simulink model "VirtualVehicleTemplate"  (R2023a)
settings: configuration reference "VehicleVariable" (kept outside this file)
StartFcn:
  | %tic
StopFcn:
  | %toc
undefined symbols (not defined in the file): CtrlEcuRevLim, CtrlTcuInitGear, CtrlVcuCltch1InitCmd, Disabled, DriverPreviewDist, EnvAbsPrs, EnvAirTemp, EnvGrvty, EnvNomFrictionScaling, EnvNominalGrade, EnvWindVelX, EnvWindVelY, EnvWindVelZ, FTP75, PlntVehDstCGFrntAxl, PlntVehDstCGRearAxl, PlntVehInitLatPos, PlntVehInitLongPos, PlntVehInitPitchAng, PlntVehInitRollAng, PlntVehInitVertPos, PlntVehInitYawAng, PlntVehMass, PlntVehTrckWdth, PlntVehYawMomentInertia, ScnCRMaxLatAccel, ScnCRRadius, ScnDLCGateLongPos, ScnDLCLatRef, ScnDLCLatRefOffset, ScnDLCLongRefBpt, ScnDLCLongRefStartPos, ScnDLCVehicleWidth, ScnFHCounterDwellTime, ScnFHInitialDwellTime, ScnFHReturnTime, ScnFHRollRateZeroCross, ScnFHSteerAmp, ScnFHSteerSpeed, ScnISHandwheelRate, ScnISMaxHandwheelAng, ScnISMaxLatAccel, ScnISSteerHoldTime, ScnLongVelRef, ScnSDDwellTime, ScnSDSteerAmp, ScnSDSteerFreq, ScnSimTime, ScnSSFinalFreq, ScnSSSteerAmp, ScnSSSweepTime, ScnStartTime
libraries: simulink x18, vehdynlibscenariocommon x7, vehdynlibviscommon x3, vehdynlibdriver x2, sim3dgroundtruthsensorlib x2, autolibshared x2, autolibsharedcommon x1, sharedtransform x1, sim3dlib x1, sim3dautolib x1
(part 2 of 5)

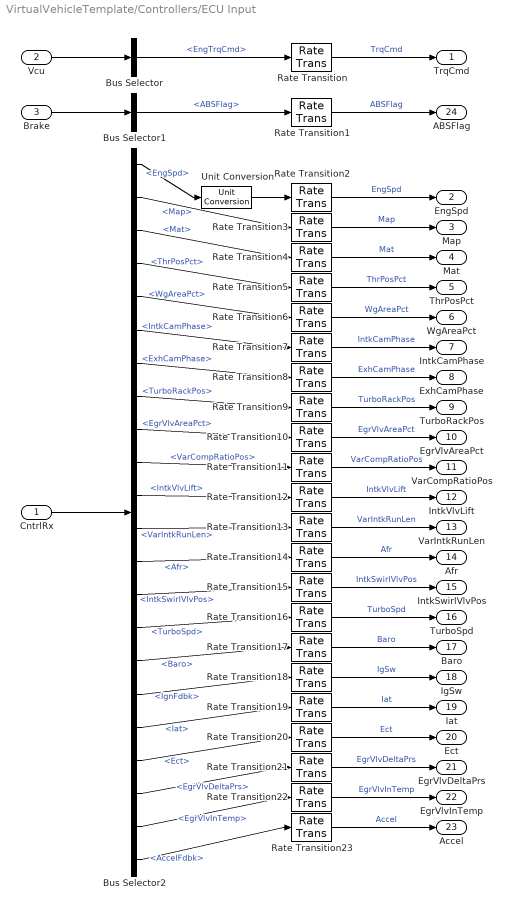
== system VirtualVehicleTemplate/Controllers/ECU Input ==
  CntrlRx : Inport
  Vcu : Inport  Port=2
  Brake : Inport  Port=3
  Bus Selector : BusSelector  OutputSignals=EngTrqCmd
  Bus Selector1 : BusSelector  OutputSignals=ABSFlag
  Bus Selector2 : BusSelector  OutputSignals=Trans.EngSpd,Engine.Map,Engine.Mat,Engine.ThrPosPct,Engine.WgAreaPct,Engine.IntkCamPhase,Engine.ExhCamPhase,Engine.TurboRackPos,Engine.EgrVlvAreaPct,Engine.VarCompRatioPos,Engine.IntkVlvLift,Engine.VarIntkRunLen,Engine.Afr,Engine.IntkSwirlVlvPos,Engine.TurboSpd,Env.Baro,Driver.IgnFdbk,Engine.Iat,Engine.Ect,Engine.EgrVlvDeltaPrs,Engine.EgrVlvInTemp,Driver.AccelFdbk
  Rate Transition{,1..23} (24 alike) : RateTransition  Deterministic=off
  Unit Conversion : UnitConversion
  TrqCmd : Outport
  EngSpd : Outport  Port=2
  Map : Outport  Port=3
  Mat : Outport  Port=4
  ThrPosPct : Outport  Port=5
  WgAreaPct : Outport  Port=6
  IntkCamPhase : Outport  Port=7
  ExhCamPhase : Outport  Port=8
  TurboRackPos : Outport  Port=9
  EgrVlvAreaPct : Outport  Port=10
  VarCompRatioPos : Outport  Port=11
  IntkVlvLift : Outport  Port=12
  VarIntkRunLen : Outport  Port=13
  Afr : Outport  Port=14
  IntkSwirlVlvPos : Outport  Port=15
  TurboSpd : Outport  Port=16
  Baro : Outport  Port=17
  IgSw : Outport  Port=18
  Iat : Outport  Port=19
  Ect : Outport  Port=20
  EgrVlvDeltaPrs : Outport  Port=21
  EgrVlvInTemp : Outport  Port=22
  Accel : Outport  Port=23
  ABSFlag : Outport  Port=24
  wires:
  Bus Selector2/13 -> Rate Transition14/1  "<Afr>"
  Bus Selector2/1 -> Unit Conversion/1  "<EngSpd>"
  Bus Selector2/21 -> Rate Transition22/1  "<EgrVlvInTemp>"
  Bus Selector2/19 -> Rate Transition20/1  "<Ect>"
  Bus Selector2/9 -> Rate Transition10/1  "<EgrVlvAreaPct>"
  Bus Selector2/15 -> Rate Transition16/1  "<TurboSpd>"
  Bus Selector2/17 -> Rate Transition18/1  "<IgnFdbk>"
  Bus Selector2/16 -> Rate Transition17/1  "<Baro>"
  Bus Selector2/2 -> Rate Transition3/1  "<Map>"
  Bus Selector2/18 -> Rate Transition19/1  "<Iat>"
  Bus Selector2/8 -> Rate Transition9/1  "<TurboRackPos>"
  Bus Selector2/10 -> Rate Transition11/1  "<VarCompRatioPos>"
  Bus Selector2/3 -> Rate Transition4/1  "<Mat>"
  Unit Conversion/1 -> Rate Transition2/1
  Bus Selector2/14 -> Rate Transition15/1  "<IntkSwirlVlvPos>"
  Bus Selector2/7 -> Rate Transition8/1  "<ExhCamPhase>"
  Bus Selector2/6 -> Rate Transition7/1  "<IntkCamPhase>"
  CntrlRx/1 -> Bus Selector2/1
  Bus Selector2/11 -> Rate Transition12/1  "<IntkVlvLift>"
  Bus Selector2/20 -> Rate Transition21/1  "<EgrVlvDeltaPrs>"
  Bus Selector2/12 -> Rate Transition13/1  "<VarIntkRunLen>"
  Bus Selector2/5 -> Rate Transition6/1  "<WgAreaPct>"
  Bus Selector2/4 -> Rate Transition5/1  "<ThrPosPct>"
  Bus Selector/1 -> Rate Transition/1  "<EngTrqCmd>"
  Vcu/1 -> Bus Selector/1
  Brake/1 -> Bus Selector1/1
  Bus Selector1/1 -> Rate Transition1/1  "<ABSFlag>"
  Bus Selector2/22 -> Rate Transition23/1  "<AccelFdbk>"
  Rate Transition/1 -> TrqCmd/1  "TrqCmd"
  Rate Transition1/1 -> ABSFlag/1  "ABSFlag"
  Rate Transition2/1 -> EngSpd/1  "EngSpd"
  Rate Transition3/1 -> Map/1  "Map"
  Rate Transition4/1 -> Mat/1  "Mat"
  Rate Transition5/1 -> ThrPosPct/1  "ThrPosPct"
  Rate Transition6/1 -> WgAreaPct/1  "WgAreaPct"
  Rate Transition7/1 -> IntkCamPhase/1  "IntkCamPhase"
  Rate Transition8/1 -> ExhCamPhase/1  "ExhCamPhase"
  Rate Transition9/1 -> TurboRackPos/1  "TurboRackPos"
  Rate Transition10/1 -> EgrVlvAreaPct/1  "EgrVlvAreaPct"
  Rate Transition11/1 -> VarCompRatioPos/1  "VarCompRatioPos"
  Rate Transition12/1 -> IntkVlvLift/1  "IntkVlvLift"
  Rate Transition13/1 -> VarIntkRunLen/1  "VarIntkRunLen"
  Rate Transition14/1 -> Afr/1  "Afr"
  Rate Transition15/1 -> IntkSwirlVlvPos/1  "IntkSwirlVlvPos"
  Rate Transition16/1 -> TurboSpd/1  "TurboSpd"
  Rate Transition17/1 -> Baro/1  "Baro"
  Rate Transition18/1 -> IgSw/1  "IgSw"
  Rate Transition19/1 -> Iat/1  "Iat"
  Rate Transition20/1 -> Ect/1  "Ect"
  Rate Transition21/1 -> EgrVlvDeltaPrs/1  "EgrVlvDeltaPrs"
  Rate Transition22/1 -> EgrVlvInTemp/1  "EgrVlvInTemp"
  Rate Transition23/1 -> Accel/1  "Accel"

== system VirtualVehicleTemplate/Controllers/ECU Output ==
  ThrPosPctCmd : Inport
  WgAreaPctCmd : Inport  Port=2
  InjPw : Inport  Port=3
  FuelMainSoi : Inport  Port=4
  SpkAdv : Inport  Port=5
  IntkCamPhaseCmd : Inport  Port=6
  ExhCamPhaseCmd : Inport  Port=7
  TurboRackPosCmd : Inport  Port=8
  EgrVlvAreaPctCmd : Inport  Port=9
  VarCompRatioPosCmd : Inport  Port=10
  IntkVlvLiftCmd : Inport  Port=11
  VarIntkRunLenCmd : Inport  Port=12
  ClsdLpFuelMult : Inport  Port=13
  IntkSwirlVlvPosCmd : Inport  Port=14
  TrqCmdISC : Inport  Port=15
  LoadCmd : Inport  Port=16
  EstIntkPortFlw : Inport  Port=17
  Bus Creator : BusCreator  Inputs=17
  Engine : Outport
  wires:
  Bus Creator/1 -> Engine/1  "Engine"
  EstIntkPortFlw/1 -> Bus Creator/17  "EstIntkPortFlw"
  ThrPosPctCmd/1 -> Bus Creator/1  "ThrPosPctCmd"
  InjPw/1 -> Bus Creator/3  "InjPw"
  SpkAdv/1 -> Bus Creator/5  "SpkAdv"
  TrqCmdISC/1 -> Bus Creator/15  "TrqCmd"
  VarCompRatioPosCmd/1 -> Bus Creator/10  "VarCompRatioPosCmd"
  FuelMainSoi/1 -> Bus Creator/4  "FuelMainSoi"
  IntkCamPhaseCmd/1 -> Bus Creator/6  "IntkCamPhaseCmd"
  ClsdLpFuelMult/1 -> Bus Creator/13  "ClsdLpFuelMult"
  WgAreaPctCmd/1 -> Bus Creator/2  "WgAreaPctCmd"
  ExhCamPhaseCmd/1 -> Bus Creator/7  "ExhCamPhaseCmd"
  TurboRackPosCmd/1 -> Bus Creator/8  "TurboRackPosCmd"
  EgrVlvAreaPctCmd/1 -> Bus Creator/9  "EgrVlvAreaPctCmd"
  IntkVlvLiftCmd/1 -> Bus Creator/11  "IntkVlvLiftCmd"
  VarIntkRunLenCmd/1 -> Bus Creator/12  "VarIntkRunLenCmd"
  IntkSwirlVlvPosCmd/1 -> Bus Creator/14  "IntkSwirlVlvPosCmd"
  LoadCmd/1 -> Bus Creator/16  "LoadCmd"

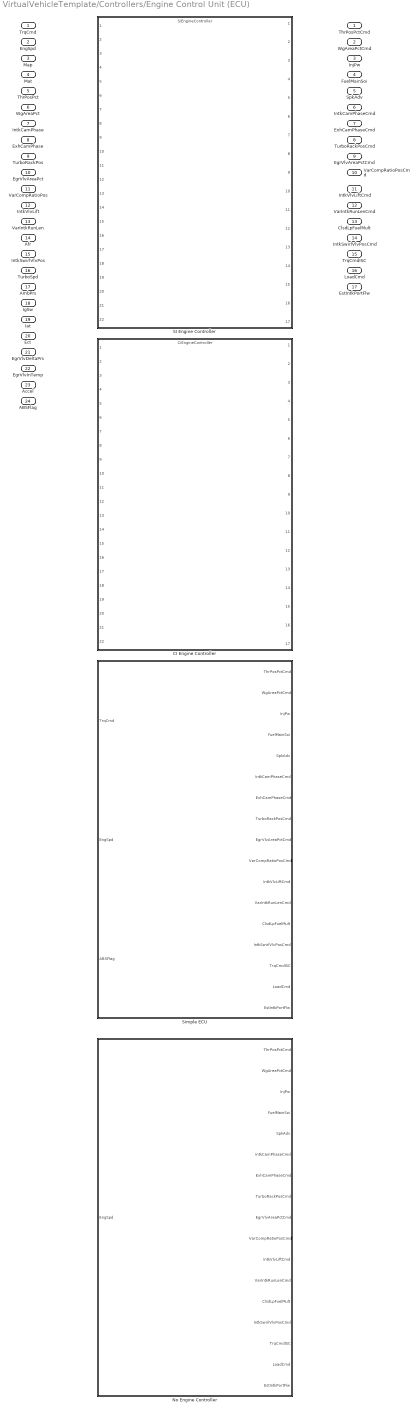
== system VirtualVehicleTemplate/Controllers/Engine Control Unit (ECU) ==
  TrqCmd : Inport
  EngSpd : Inport  Port=2
  Map : Inport  Port=3
  Mat : Inport  Port=4
  ThrPosPct : Inport  Port=5
  WgAreaPct : Inport  Port=6
  IntkCamPhase : Inport  Port=7
  ExhCamPhase : Inport  Port=8
  TurboRackPos : Inport  Port=9
  EgrVlvAreaPct : Inport  Port=10
  VarCompRatioPos : Inport  Port=11
  IntkVlvLift : Inport  Port=12
  VarIntkRunLen : Inport  Port=13
  Afr : Inport  Port=14
  IntkSwirlVlvPos : Inport  Port=15
  TurboSpd : Inport  Port=16
  AmbPrs : Inport  Port=17
  IgSw : Inport  Port=18
  Iat : Inport  Port=19
  Ect : Inport  Port=20
  EgrVlvDeltaPrs : Inport  Port=21
  EgrVlvInTemp : Inport  Port=22
  Accel : Inport  Port=23
  ABSFlag : Inport  Port=24
  CI Engine Controller : ModelReference  ModelNameDialog=CiEngineController  SimulationMode=Normal  VariantControl=CI Engine Controller  ModelReferenceVersion=7.0
  No Engine Controller : Subsystem  VariantControl=No Engine Controller
  SI Engine Controller : ModelReference  ModelNameDialog=SiEngineController  SimulationMode=Normal  VariantControl=SI Engine Controller  ModelReferenceVersion=6.2
  Simple ECU : Subsystem  VariantControl=Simple ECU
  ThrPosPctCmd : Outport  VectorParamsAs1DForOutWhenUnconnected=off
  WgAreaPctCmd : Outport  Port=2  VectorParamsAs1DForOutWhenUnconnected=off
  InjPw : Outport  Port=3  VectorParamsAs1DForOutWhenUnconnected=off
  FuelMainSoi : Outport  Port=4  VectorParamsAs1DForOutWhenUnconnected=off
  SpkAdv : Outport  Port=5  VectorParamsAs1DForOutWhenUnconnected=off
  IntkCamPhaseCmd : Outport  Port=6  VectorParamsAs1DForOutWhenUnconnected=off
  ExhCamPhaseCmd : Outport  Port=7  VectorParamsAs1DForOutWhenUnconnected=off
  TurboRackPosCmd : Outport  Port=8  VectorParamsAs1DForOutWhenUnconnected=off
  EgrVlvAreaPctCmd : Outport  Port=9  VectorParamsAs1DForOutWhenUnconnected=off
  VarCompRatioPosCmd : Outport  Port=10  VectorParamsAs1DForOutWhenUnconnected=off
  IntkVlvLiftCmd : Outport  Port=11  VectorParamsAs1DForOutWhenUnconnected=off
  VarIntkRunLenCmd : Outport  Port=12  VectorParamsAs1DForOutWhenUnconnected=off
  ClsdLpFuelMult : Outport  Port=13  VectorParamsAs1DForOutWhenUnconnected=off
  IntkSwirlVlvPosCmd : Outport  Port=14  VectorParamsAs1DForOutWhenUnconnected=off
  TrqCmdISC : Outport  Port=15  VectorParamsAs1DForOutWhenUnconnected=off
  LoadCmd : Outport  Port=16  VectorParamsAs1DForOutWhenUnconnected=off
  EstIntkPortFlw : Outport  Port=17  VectorParamsAs1DForOutWhenUnconnected=off

== system VirtualVehicleTemplate/Controllers/TCU Input ==
  CntrlRx : Inport
  Brake : Inport  Port=2
  Bus Selector : BusSelector  OutputSignals=ABSFlag
  Bus Selector1 : BusSelector  OutputSignals=Driver.AccelFdbk,Driver.DecelFdbk,Driver.GearFdbk,Trans.EngSpd,Wheels.Omega,Vehicle
  Ground : Ground
  Ground1 : Ground
  Rate Transition{1..8,23} (9 alike) : RateTransition  Deterministic=off
  <AccFdbk> : Outport
  <DecelFdbk> : Outport  Port=2
  <GearFdbk> : Outport  Port=3
  <EngSpd> : Outport  Port=4
  <Omega> : Outport  Port=5
  <Vehicle> : Outport  Port=6
  ABSFlag : Outport  Port=7
  UpReq : Outport  Port=8
  DnReq : Outport  Port=9
  wires:
  Bus Selector1/6 -> Rate Transition5/1  "<Vehicle>"
  Bus Selector1/2 -> Rate Transition1/1  "<DecelFdbk>"
  Ground/1 -> Rate Transition7/1
  CntrlRx/1 -> Bus Selector1/1
  Bus Selector1/1 -> Rate Transition23/1  "<AccelFdbk>"
  Bus Selector1/5 -> Rate Transition4/1  "<Omega>"
  Bus Selector1/4 -> Rate Transition3/1  "<EngSpd>"
  Bus Selector1/3 -> Rate Transition2/1  "<GearFdbk>"
  Ground1/1 -> Rate Transition8/1
  Bus Selector/1 -> Rate Transition6/1  "<ABSFlag>"
  Brake/1 -> Bus Selector/1
  Rate Transition23/1 -> <AccFdbk>/1
  Rate Transition1/1 -> <DecelFdbk>/1
  Rate Transition2/1 -> <GearFdbk>/1
  Rate Transition3/1 -> <EngSpd>/1
  Rate Transition4/1 -> <Omega>/1
  Rate Transition5/1 -> <Vehicle>/1
  Rate Transition6/1 -> ABSFlag/1
  Rate Transition7/1 -> UpReq/1
  Rate Transition8/1 -> DnReq/1

== system VirtualVehicleTemplate/Controllers/TCU Output ==
  GearCmd : Inport
  Bus Creator1 : BusCreator  Inputs=1
  Trans : Outport
  wires:
  Bus Creator1/1 -> Trans/1  "Trans"
  GearCmd/1 -> Bus Creator1/1  "GearCmd"

== system VirtualVehicleTemplate/Controllers/Transmission Control Unit (TCU) ==
  Accel : Inport
  BrkCmd : Inport  Port=2
  GearReq : Inport  Port=3
  EngSpd : Inport  Port=4
  Omega : Inport  Port=5  Unit=rad/s
  VehSpdFdbk : Inport  Port=6
  ABSFlag : Inport  Port=7
  UpReq : Inport  Port=8
  DownReq : Inport  Port=9  Unit=rad/s
  Driver Pass Through : ModelReference  ModelNameDialog=DriverPassThrough.slx  VariantControl=Driver Pass Through  ModelReferenceVersion=6.0
  Transmission Controller : ModelReference  ModelNameDialog=TransmissionController  VariantControl=PRNDL Controller  ModelReferenceVersion=6.0
  " Gear" : Outport  VectorParamsAs1DForOutWhenUnconnected=off

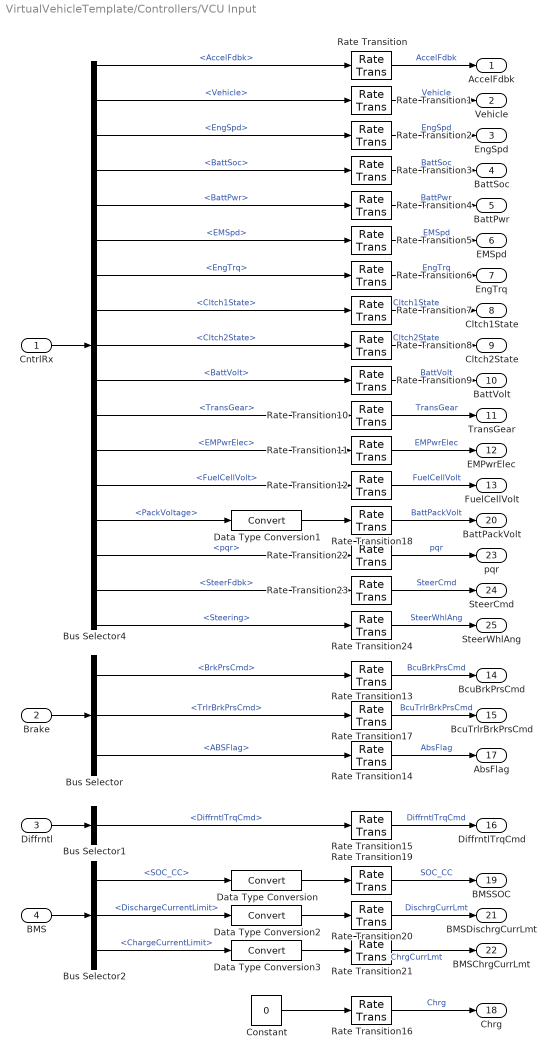
== system VirtualVehicleTemplate/Controllers/VCU Input ==
  CntrlRx : Inport
  Brake : Inport  Port=2
  Diffrntl : Inport  Port=3
  BMS : Inport  Port=4
  Bus Selector : BusSelector  OutputSignals=BrkPrsCmd,TrlrBrkPrsCmd,ABSFlag
  Bus Selector1 : BusSelector  OutputSignals=DiffrntlTrqCmd
  Bus Selector2 : BusSelector  OutputSignals=BMSInfo.SOC.SOC_CC,BMSCmd.CurrentLimitsBus.DischargeCurrentLimit,BMSCmd.CurrentLimitsBus.ChargeCurrentLimit
  Bus Selector4 : BusSelector  OutputSignals=Driver.AccelFdbk,Vehicle,Trans.EngSpd,Battery.BattSoc,Battery.BattPwr,Trans.EMSpd,Engine.EngTrq,Trans.Cltch1State,Trans.Cltch2State,Battery.BattVolt,Trans.TransGear,EM.EMPwrElec,FuelCell.FuelCellVolt,Battery.BMSSensors.PackVoltage,IMU.pqr,Driver.SteerFdbk,Steering
  Constant : Constant  Value=0  SampleTime=-1
  Data Type Conversion{,1..3} (4 alike) : DataTypeConversion  SaturateOnIntegerOverflow=off  RndMeth=Floor
  Rate Transition{,1..24} (25 alike) : RateTransition  Deterministic=off
  AccelFdbk : Outport
  Vehicle : Outport  Port=2
  EngSpd : Outport  Port=3
  BattSoc : Outport  Port=4
  BattPwr : Outport  Port=5
  EMSpd : Outport  Port=6
  EngTrq : Outport  Port=7
  Cltch1State : Outport  Port=8
  Cltch2State : Outport  Port=9
  BattVolt : Outport  Port=10
  TransGear : Outport  Port=11
  EMPwrElec : Outport  Port=12
  FuelCellVolt : Outport  Port=13
  BcuBrkPrsCmd : Outport  Port=14
  BcuTrlrBrkPrsCmd : Outport  Port=15
  DiffrntlTrqCmd : Outport  Port=16
  AbsFlag : Outport  Port=17
  Chrg : Outport  Port=18
  BMSSOC : Outport  Port=19
  BattPackVolt : Outport  Port=20
  BMSDischrgCurrLmt : Outport  Port=21
  BMSChrgCurrLmt : Outport  Port=22
  pqr : Outport  Port=23
  SteerCmd : Outport  Port=24
  SteerWhlAng : Outport  Port=25
  wires:
  Bus Selector4/5 -> Rate Transition4/1  "<BattPwr>"
  Bus Selector4/1 -> Rate Transition/1  "<AccelFdbk>"
  Bus Selector4/7 -> Rate Transition6/1  "<EngTrq>"
  Bus Selector4/4 -> Rate Transition3/1  "<BattSoc>"
  Bus Selector4/6 -> Rate Transition5/1  "<EMSpd>"
  CntrlRx/1 -> Bus Selector4/1
  Bus Selector4/11 -> Rate Transition10/1  "<TransGear>"
  Bus Selector4/9 -> Rate Transition8/1  "<Cltch2State>"
  Bus Selector4/13 -> Rate Transition12/1  "<FuelCellVolt>"
  Bus Selector4/2 -> Rate Transition1/1  "<Vehicle>"
  Bus Selector4/8 -> Rate Transition7/1  "<Cltch1State>"
  Bus Selector4/10 -> Rate Transition9/1  "<BattVolt>"
  Bus Selector4/3 -> Rate Transition2/1  "<EngSpd>"
  Bus Selector4/12 -> Rate Transition11/1  "<EMPwrElec>"
  Bus Selector/1 -> Rate Transition13/1  "<BrkPrsCmd>"
  Constant/1 -> Rate Transition16/1
  Brake/1 -> Bus Selector/1
  Bus Selector/3 -> Rate Transition14/1  "<ABSFlag>"
  Diffrntl/1 -> Bus Selector1/1
  Bus Selector1/1 -> Rate Transition15/1  "<DiffrntlTrqCmd>"
  Rate Transition/1 -> AccelFdbk/1  "AccelFdbk"
  Rate Transition1/1 -> Vehicle/1  "Vehicle"
  Rate Transition2/1 -> EngSpd/1  "EngSpd"
  Rate Transition3/1 -> BattSoc/1  "BattSoc"
  Rate Transition4/1 -> BattPwr/1  "BattPwr"
  Rate Transition5/1 -> EMSpd/1  "EMSpd"
  Rate Transition6/1 -> EngTrq/1  "EngTrq"
  Rate Transition7/1 -> Cltch1State/1  "Cltch1State"
  Rate Transition8/1 -> Cltch2State/1  "Cltch2State"
  Rate Transition9/1 -> BattVolt/1  "BattVolt"
  Rate Transition10/1 -> TransGear/1  "TransGear"
  Rate Transition11/1 -> EMPwrElec/1  "EMPwrElec"
  Rate Transition12/1 -> FuelCellVolt/1  "FuelCellVolt"
  Rate Transition13/1 -> BcuBrkPrsCmd/1  "BcuBrkPrsCmd"
  Rate Transition14/1 -> AbsFlag/1  "AbsFlag"
  Rate Transition15/1 -> DiffrntlTrqCmd/1  "DiffrntlTrqCmd"
  Rate Transition16/1 -> Chrg/1  "Chrg"
  Rate Transition20/1 -> BMSDischrgCurrLmt/1  "DischrgCurrLmt"
  Rate Transition19/1 -> BMSSOC/1  "SOC_CC"
  Rate Transition21/1 -> BMSChrgCurrLmt/1  "ChrgCurrLmt"
  Data Type Conversion3/1 -> Rate Transition21/1
  Data Type Conversion2/1 -> Rate Transition20/1
  Bus Selector2/1 -> Data Type Conversion/1  "<SOC_CC>"
  Data Type Conversion/1 -> Rate Transition19/1
  Bus Selector2/3 -> Data Type Conversion3/1  "<ChargeCurrentLimit>"
  Bus Selector2/2 -> Data Type Conversion2/1  "<DischargeCurrentLimit>"
  BMS/1 -> Bus Selector2/1
  Data Type Conversion1/1 -> Rate Transition18/1
  Rate Transition18/1 -> BattPackVolt/1  "BattPackVolt"
  Bus Selector4/14 -> Data Type Conversion1/1  "<PackVoltage>"
  Bus Selector/2 -> Rate Transition17/1  "<TrlrBrkPrsCmd>"
  Rate Transition17/1 -> BcuTrlrBrkPrsCmd/1  "BcuTrlrBrkPrsCmd"
  Rate Transition22/1 -> pqr/1  "pqr"
  Rate Transition23/1 -> SteerCmd/1  "SteerCmd"
  Rate Transition24/1 -> SteerWhlAng/1  "SteerWhlAng"
  Bus Selector4/15 -> Rate Transition22/1  "<pqr>"
  Bus Selector4/16 -> Rate Transition23/1  "<SteerFdbk>"
  Bus Selector4/17 -> Rate Transition24/1  "<Steering>"

== system VirtualVehicleTemplate/Controllers/VCU Output ==
  EngTrqCmd : Inport
  EMTrqCmd : Inport  Port=2
  VcuBrkPrsCmd : Inport  Port=3
  VcuTrlrBrkPrsCmd : Inport  Port=4
  Cltch1Cmd : Inport  Port=5
  Neutral : Inport  Port=6
  FuelCellCurrCmd : Inport  Port=7
  FuelCellTempCmd : Inport  Port=8
  Bus Creator5 : BusCreator  Inputs=8
  Vcu : Outport
  wires:
  Cltch1Cmd/1 -> Bus Creator5/5  "Cltch1Cmd"
  EngTrqCmd/1 -> Bus Creator5/1  "EngTrqCmd"
  Bus Creator5/1 -> Vcu/1  "Vcu"
  VcuBrkPrsCmd/1 -> Bus Creator5/3  "VcuBrkPrsCmd"
  Neutral/1 -> Bus Creator5/6  "Neutral"
  FuelCellCurrCmd/1 -> Bus Creator5/7  "FuelCellCurrCmd"
  EMTrqCmd/1 -> Bus Creator5/2  "EMTrqCmd"
  FuelCellTempCmd/1 -> Bus Creator5/8  "FuelCellTempCmd"
  VcuTrlrBrkPrsCmd/1 -> Bus Creator5/4  "VcuTrlrBrkPrsCmd"

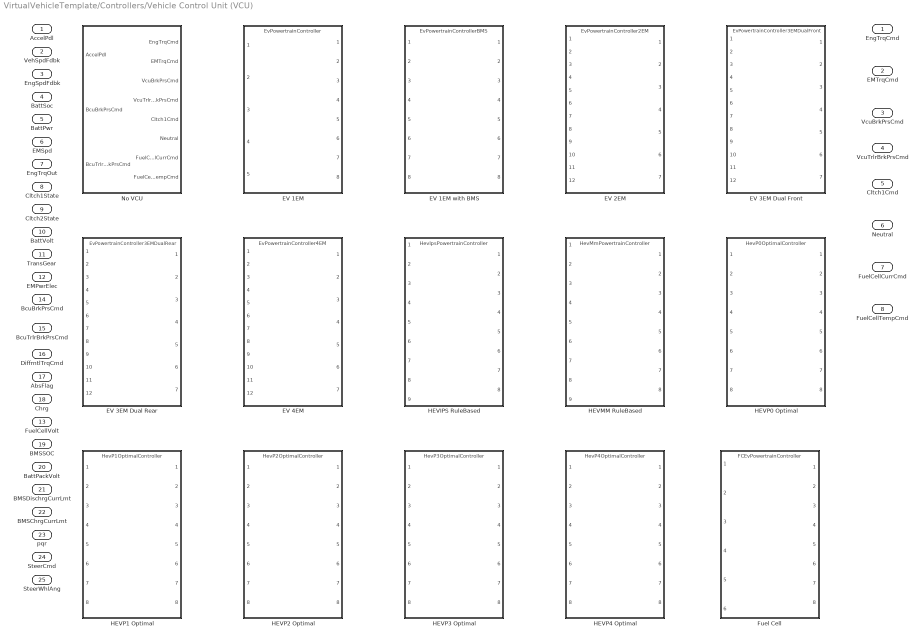
== system VirtualVehicleTemplate/Controllers/Vehicle Control Unit (VCU) ==
  AccelPdl : Inport
  VehSpdFdbk : Inport  Port=2
  EngSpdFdbk : Inport  Port=3
  BattSoc : Inport  Port=4
  BattPwr : Inport  Port=5
  EMSpd : Inport  Port=6
  EngTrqOut : Inport  Port=7
  Cltch1State : Inport  Port=8
  Cltch2State : Inport  Port=9
  BattVolt : Inport  Port=10
  TransGear : Inport  Port=11
  EMPwrElec : Inport  Port=12
  FuelCellVolt : Inport  Port=13
  BcuBrkPrsCmd : Inport  Port=14
  BcuTrlrBrkPrsCmd : Inport  Port=15
  DiffrntlTrqCmd : Inport  Port=16
  AbsFlag : Inport  Port=17
  Chrg : Inport  Port=18
  BMSSOC : Inport  Port=19
  BattPackVolt : Inport  Port=20
  BMSDischrgCurrLmt : Inport  Port=21
  BMSChrgCurrLmt : Inport  Port=22
  pqr : Inport  Port=23
  SteerCmd : Inport  Port=24
  SteerWhlAng : Inport  Port=25
  EV 1EM : ModelReference  ModelNameDialog=EvPowertrainController  VariantControl=EV 1EM  ModelReferenceVersion=6.24
  EV 1EM with BMS : ModelReference  ModelNameDialog=EvPowertrainControllerBMS.slx  VariantControl=EV 1EM with BMS  ModelReferenceVersion=6.17
  EV 2EM : ModelReference  ModelNameDialog=EvPowertrainController2EM.slx  VariantControl=EV 2EM  ModelReferenceVersion=6.43
  EV 3EM Dual Front : ModelReference  ModelNameDialog=EvPowertrainController3EMDualFront.slx  VariantControl=EV 3EM Dual Front  ModelReferenceVersion=6.44
  EV 3EM Dual Rear : ModelReference  ModelNameDialog=EvPowertrainController3EMDualRear.slx  VariantControl=EV 3EM Dual Rear  ModelReferenceVersion=6.43
  EV 4EM : ModelReference  ModelNameDialog=EvPowertrainController4EM.slx  VariantControl=EV 4EM  ModelReferenceVersion=6.46
  Fuel Cell : ModelReference  ModelNameDialog=FCEvPowertrainController  VariantControl=Fuel Cell  ModelReferenceVersion=6.12
  HEVIPS RuleBased : ModelReference  ModelNameDialog=HevIpsPowertrainController  VariantControl=HEVIPS RuleBased  ModelReferenceVersion=11.16
  HEVMM RuleBased : ModelReference  ModelNameDialog=HevMmPowertrainController  VariantControl=HEVMM RuleBased  ModelReferenceVersion=11.15
  HEVP0 Optimal : ModelReference  ModelNameDialog=HevP0OptimalController  VariantControl=HEVP0 Optimal  ModelReferenceVersion=6.17
  HEVP1 Optimal : ModelReference  ModelNameDialog=HevP1OptimalController  VariantControl=HEVP1 Optimal  ModelReferenceVersion=6.13
  HEVP2 Optimal : ModelReference  ModelNameDialog=HevP2OptimalController  VariantControl=HEVP2 Optimal  ModelReferenceVersion=6.14
  HEVP3 Optimal : ModelReference  ModelNameDialog=HevP3OptimalController  VariantControl=HEVP3 Optimal  ModelReferenceVersion=6.13
  HEVP4 Optimal : ModelReference  ModelNameDialog=HevP4OptimalController  VariantControl=HEVP4 Optimal  ModelReferenceVersion=6.13
  No VCU : Subsystem  SystemSampleTime=.01  VariantControl=No VCU
  EngTrqCmd : Outport  VectorParamsAs1DForOutWhenUnconnected=off
  EMTrqCmd : Outport  Port=2  VectorParamsAs1DForOutWhenUnconnected=off
  VcuBrkPrsCmd : Outport  Port=3  VectorParamsAs1DForOutWhenUnconnected=off
  VcuTrlrBrkPrsCmd : Outport  Port=4  VectorParamsAs1DForOutWhenUnconnected=off
  Cltch1Cmd : Outport  Port=5  VectorParamsAs1DForOutWhenUnconnected=off
  Neutral : Outport  Port=6  VectorParamsAs1DForOutWhenUnconnected=off
  FuelCellCurrCmd : Outport  Port=7  VectorParamsAs1DForOutWhenUnconnected=off
  FuelCellTempCmd : Outport  Port=8  VectorParamsAs1DForOutWhenUnconnected=off

== system VirtualVehicleTemplate/Driver Commands/Driver Commands ==
  VehRef : Inport
  VehFdbk : Inport  Port=2
  Env : Inport  Port=3
  SteerCmd : Inport  Port=4
  AccelCmd : Inport  Port=5
  BrakeCmd : Inport  Port=6
  GearCmd : Inport  Port=7
  Longitudinal Driver : Subsystem  VariantControl=driverType==1
  Open Loop : Subsystem  VariantControl=driverType==4
  Predictive Driver : Subsystem  VariantControl=driverType==2
  Predictive Stanley Driver : Subsystem  VariantControl=driverType==3
  " Driver" : Outport  VectorParamsAs1DForOutWhenUnconnected=off

== system VirtualVehicleTemplate/Environment/Estimated Grade ==
  Gnd : Inport
  Atan : Trigonometry  Operator=atan
  Bus Selector : BusSelector  OutputSignals=z  OutputAsBus=on
  Bus to Vector : BusToVector
  Constant Grade : Constant  Value=EnvNominalGrade  SampleTime=-1
  Constant1 : Constant  Value=PlntVehDstCGFrntAxl+PlntVehDstCGRearAxl  SampleTime=-1
  Divide : Product  Inputs=*/
  Gain : Gain  Gain=.5
  Gain1 : Gain  Gain=.5
  Grade Source : ManualSwitch  CurrentSetting=0
  Selector : Selector  InputPortWidth=4  IndexOptions=Index vector (dialog)  Indices=[1 2]  OutputSizes=1
  Selector1 : Selector  InputPortWidth=4  IndexOptions=Index vector (dialog)  Indices=[3 4]  OutputSizes=1
  Signal Specification : SignalSpecification  Unit=rad
  Signal Specification1 : SignalSpecification  Unit=deg
  Signal Specification2 : SignalSpecification  Unit=deg
  Subtract : Sum  Inputs=+-
  Sum of Elements : Sum  Inputs=+
  Sum of Elements1 : Sum  Inputs=+
  Unit Conversion : UnitConversion
  Grade : Outport  PortDimensions=1
  wires:
  Divide/1 -> Atan/1
  Bus Selector/1 -> Bus to Vector/1
  Sum of Elements/1 -> Gain/1
  Gain/1 -> Subtract/1
  Selector/1 -> Sum of Elements/1
  Sum of Elements1/1 -> Gain1/1
  Signal Specification/1 -> Unit Conversion/1
  Constant1/1 -> Divide/2
  Selector1/1 -> Sum of Elements1/1
  Gain1/1 -> Subtract/2
  Subtract/1 -> Divide/1
  Atan/1 -> Signal Specification/1
  Grade Source/1 -> Grade/1  "Grade"
  Gnd/1 -> Bus Selector/1
  Bus to Vector/1 -> Selector1/1, Selector/1
  Constant Grade/1 -> Signal Specification2/1
  Signal Specification2/1 -> Grade Source/2
  Unit Conversion/1 -> Signal Specification1/1
  Signal Specification1/1 -> Grade Source/1  "Grade"

== system VirtualVehicleTemplate/Environment/Ground Feedback ==
  Friction : Inport
  WheelFdbk : Inport  Port=2
  3D Engine : Subsystem  VariantControl=1
  Constant : Subsystem  VariantControl=0
  Ground : Outport  VectorParamsAs1DForOutWhenUnconnected=off

== system VirtualVehicleTemplate/Environment/Varying Friction ==
  In1 : Inport
  In2 : Inport  Port=2
  Cg : Inport  Port=3
  Constant Friction : Subsystem  VariantControl=0
  Varying Friction : Subsystem  VariantControl=1
  FricCoeffLambda : Outport

== system VirtualVehicleTemplate/Scenarios/Drive Cycle ==
  "VehFdbk " : Inport
  Bus Creator : BusCreator  Inputs=3
  Bus Creator1 : BusCreator  Inputs=16
  Constant{,2..3,8,13..15,17} (8 alike) : Constant  Value=0
  Constant{1,4..7,9..12} (9 alike) : Constant  Value=false
  Constant16 : Constant  Value=zeros(1,3)
  Drive Cycle Source : autolibshared/Drive Cycle Source  cycleVar=FTP75  fileVar=L:\Bauto\matlab\test\toolbox\shared\autoblks\scenario\adac.txt  tfinal="2474  seconds"  cycleRepeat=off  outAccPort=off  outGearPort=off  gearList=No gear data  t_wot1=1  xdot_woto=0  xdot_wot1=26.8  t_wot2=30  xdot_wot2=0  t_wotend=40  srcUnit=m/s  outUnit=mph  srcAccUnit=m/s/s  outAccUnit=m/s^2  dt=0  aMode=6  faultOption=off  velBnd=2  velBndUnit=mph  inUnit=m/s  timeBnd=1  failOption=off  stopSim=off  maxFaultCnt=10  maxFaultTime=2  maxTotFaultTime=15  traceOption=off  dtTrace=1  traceWindow=10  lastDCname=FTP75  lastOutUnit=mph  lastDT=0  lastTB=1  lastSB=2  forceCalcBound=off
  Signal Specification : SignalSpecification  Unit=rad
  Signal Specification1 : SignalSpecification  Unit=one
  Signal Specification2 : SignalSpecification  Unit=one
  " Vis" : Outport  VectorParamsAs1DForOutWhenUnconnected=off
  " Ref" : Outport  Port=2  VectorParamsAs1DForOutWhenUnconnected=off
  " Fdbk" : Outport  Port=3  VectorParamsAs1DForOutWhenUnconnected=off
  wires:
  Constant2/1 -> Signal Specification2/1
  Constant8/1 -> Signal Specification1/1
  Constant4/1 -> Bus Creator1/7  "SteerHld"
  Signal Specification2/1 -> Bus Creator1/14  "DecelOvrCmd"
  Constant12/1 -> Bus Creator1/16  "DecelZero"
  Constant6/1 -> Bus Creator1/9  "EnblAccelOvr"
  Constant7/1 -> Bus Creator1/11  "AccelHld"
  Constant9/1 -> Bus Creator1/12  "AccelZero"
  Signal Specification1/1 -> Bus Creator1/10  "AccelOvrCmd"
  Constant11/1 -> Bus Creator1/15  "DecelHld"
  Constant10/1 -> Bus Creator1/13  "EnblDecelCmd"
  Constant5/1 -> Bus Creator1/8  "SteerZero"
  Signal Specification/1 -> Bus Creator1/6  "SteerOvrCmd"
  Constant3/1 -> Signal Specification/1
  Constant1/1 -> Bus Creator1/5  "EnblSteerCmd"
  Constant/1 -> Bus Creator1/2  "LtrlRef"
  Drive Cycle Source/1 -> Bus Creator1/1  "LngRef"
  Bus Creator1/1 -> " Ref"/1
  "VehFdbk "/1 -> " Fdbk"/1
  Bus Creator/1 -> " Vis"/1
  Constant15/1 -> Bus Creator/3  "ZRef"
  Constant14/1 -> Bus Creator/2  "YRef"
  Constant13/1 -> Bus Creator/1  "XRef"
  Constant16/1 -> Bus Creator1/3  "PoseRef"
  Constant17/1 -> Bus Creator1/4  "CurvRef"

== system VirtualVehicleTemplate/Scenarios/Reference Generator ==
  "VehFdbk " : Inport
  3D Engine : Subsystem  Variant=on  mask(3D Engine){engine3D=Disabled, SceneDesc=Open surface, dt3D=dt3D, defaultPos=Recommended for scene, X_o=X_o, Y_o=Y_o, Z_o=Z_o, phi_o=phi_o, theta_o=theta_o, psi_o=psi_o}
      mask prompts: engine3D "3D Engine"; SceneDesc "shared_sim3dblks:sim3dblkConfig:SceneDesc"; dt3D "Engine frame rate, dt3D [s]:"; X_o "Initial longitudinal position, X_o [m]:"; Y_o "Initial lateral position, Y_o [m]:"; Z_o "Initial vertical position, Z_o [m]:"; phi_o "Initial roll angle, phi_o [rad]:"; theta_o "Initial pitch angle, theta_o [rad]:"; psi_o "Initial yaw angle, psi_o [rad]:"
      mask help: This subsystem contains the interface blocks which permit the display of the vehicle in the 3D virtual environment. Enable it to view the simulation progress, disable it to inhibit the display.
      mask init:
      | GrndFdbkPath = [bdroot(gcb) '/Environment/Ground Feedback'];
      | switch get_param(gcb,'engine3D')    
      |     case 'Disabled'
      |         try
      |             set_param(GrndFdbkPath,'LabelModeActiveChoice','0');
      |             set_param([bdroot(gcb) '/Scenarios/Reference Generator/Reference Generator/Double Lane Change/Double Lane Change'],'use3DCones','off');
      |             set_param([bdroot(gcb) '/Scenarios/Reference Generator/Reference Generator/Constant Radius'],'use3DCones','off');
      |         catch
      |             disp('Warning: Ground feedback source subsystem was not found. Ground feedback source remains unchanged.');
      |         end
      |     case 'Enabled'
      |         try
      |             set_param(GrndFdbkPath,'LabelModeActiveChoice','1'); 
      |             set_param([bdroot(gcb) '/Scenarios/Reference Generator/Reference Generator/Double Lane Change/Double Lane Change'],'use3DCones','on');
      |             set_param([bdroot(gcb) '/Scenarios/Reference Generator/Reference Generator/Constant Radius'],'use3DCones','on');
      |         catch
      |             disp('Warning: Ground feedback source subsystem was not found. Ground feedback source remains unchanged.');
      |         end
      |     otherwise
      | end
      settings: AttributesFormatString=|
      | %<SceneDesc>
      | %<engine3D>
      mask Help: eval('vdynblkshelp(''vdynblks3dengine'')');
      mask TypeOptions engine3D: vdynblks:vehdynRefApp3DEng:blkRdBt_engine3D_c2 | vdynblks:vehdynRefApp3DEng:blkRdBt_engine3D_c1
      mask TypeOptions SceneDesc: 3D Engine/Simulation 3D Scene Configuration/SceneDesc
      mask Callback SceneDesc: [~] = vdynblks3Dsceneconfig(gcb);
      mask TypeOptions defaultPos: vdynblks:vehdynRefApp3DEng:blkRdBt_defaultPos_c1 | vdynblks:vehdynRefApp3DEng:blkRdBt_defaultPos_c2
      mask DialogControl engineConfig Prompt: 3D Engine Settings
      mask DialogControl SceneDesc Prompt: Scene name:
      mask DialogControl posSetup Prompt: Initial vehicle position
      mask DialogControl posSetupDesc Prompt: To use these initial vehicle positions, first Apply the initial values and then click Update the model workspaces with the initial values.
      mask DialogControl setModelPos Prompt: Update model workspaces with initial values
      mask DialogControl setModelPos Callback: [~] = vdynblksmdlWSconfig(gcb);
      mask Display: disp('3D Engine')
  Reference Generator : Subsystem  Variant=on  VariantControlMode=label  VariantControl=Variant1  LabelModeActiveChoice=Drive Cycle
  " Vis" : Outport  VectorParamsAs1DForOutWhenUnconnected=off
  " Ref" : Outport  Port=2  VectorParamsAs1DForOutWhenUnconnected=off
  " Fdbk" : Outport  Port=3  VectorParamsAs1DForOutWhenUnconnected=off
  wires:
  Reference Generator/3(" Fdbk") -> " Fdbk"/1
  Reference Generator/2(" Ref") -> " Ref"/1
  Reference Generator/1(" Vis") -> " Vis"/1
  "VehFdbk "/1 -> Reference Generator/1("VehFdbk "), 3D Engine/1(VehFdbk)

== system VirtualVehicleTemplate/Vehicle/Chassis Input ==
  Env : Inport
  Driver : Inport  Port=2
  Cntrl : Inport  Port=3
  Bus Selector1 : BusSelector  OutputSignals=Gnd.z.G_FL_z,Gnd.z.G_FR_z,Gnd.z.G_RL_z,Gnd.z.G_RR_z
  Bus Selector2 : BusSelector  OutputSignals=Wind
  Bus Selector3 : BusSelector  OutputSignals=Gnd.mu.mu_FL,Gnd.mu.mu_FR,Gnd.mu.mu_RL,Gnd.mu.mu_RR
  Bus Selector4 : BusSelector  OutputSignals=Grade
  Bus Selector5 : BusSelector  OutputSignals=SteerCmd
  Bus Selector6 : BusSelector  OutputSignals=Vcu.VcuBrkPrsCmd
  Bus Selector7 : BusSelector  OutputSignals=Gnd.DCM
  First Order Hold1 : FirstOrderHold  ErrorTolerance=inf
  Vector Concatenate : Concatenate  NumInputs=4
  Vector Concatenate1 : Concatenate  NumInputs=4
  Wind : Outport  VectorParamsAs1DForOutWhenUnconnected=off
  Gnd : Outport  Port=2  VectorParamsAs1DForOutWhenUnconnected=off
  Mu : Outport  Port=3  VectorParamsAs1DForOutWhenUnconnected=off
  Grade : Outport  Port=4  VectorParamsAs1DForOutWhenUnconnected=off
  GndDCM : Outport  Port=5  VectorParamsAs1DForOutWhenUnconnected=off
  SteerCmd : Outport  Port=6  VectorParamsAs1DForOutWhenUnconnected=off
  BrkPrsCmd : Outport  Port=7  VectorParamsAs1DForOutWhenUnconnected=off
  wires:
  Env/1 -> Bus Selector7/1, Bus Selector4/1, Bus Selector3/1, Bus Selector1/1, Bus Selector2/1
  Bus Selector2/1 -> Wind/1  "<Wind>"
  Bus Selector3/1 -> Vector Concatenate/1  "<mu_FL>"
  Bus Selector3/2 -> Vector Concatenate/2  "<mu_FR>"
  Bus Selector3/3 -> Vector Concatenate/3  "<mu_RL>"
  Bus Selector3/4 -> Vector Concatenate/4  "<mu_RR>"
  Vector Concatenate/1 -> Mu/1
  Bus Selector1/1 -> Vector Concatenate1/1  "<G_FL_z>"
  Bus Selector1/2 -> Vector Concatenate1/2  "<G_FR_z>"
  Bus Selector1/3 -> Vector Concatenate1/3  "<G_RL_z>"
  Bus Selector1/4 -> Vector Concatenate1/4  "<G_RR_z>"
  Vector Concatenate1/1 -> Gnd/1
  Driver/1 -> Bus Selector5/1
  Bus Selector5/1 -> SteerCmd/1  "<SteerCmd>"
  Cntrl/1 -> Bus Selector6/1
  Bus Selector6/1 -> First Order Hold1/1  "<VcuBrkPrsCmd>"
  Bus Selector4/1 -> Grade/1  "<Grade>"
  First Order Hold1/1 -> BrkPrsCmd/1
  Bus Selector7/1 -> GndDCM/1  "<DCM>"

== system VirtualVehicleTemplate/Vehicle/Chassis Output ==
  Veh : Inport
  Wheels : Inport  Port=2
  Steering : Inport  Port=3
  Susp : Inport  Port=4
  Out Bus Element4 : Outport  PortName=VehFdbk
  Out Bus Element1 : Outport  Port=2  PortName=WheelsFdbk
  Out Bus Element2 : Outport  Port=3  PortName=SteeringFdbk
  Out Bus Element3 : Outport  Port=4  PortName=SuspensionFdbk
  wires:
  Veh/1 -> Out Bus Element4/1
  Wheels/1 -> Out Bus Element1/1
  Steering/1 -> Out Bus Element2/1
  Susp/1 -> Out Bus Element3/1

== system VirtualVehicleTemplate/Vehicle/Drivetrain Input ==
  Cntrl : Inport
  Bus Selector3 : BusSelector  OutputSignals=Trans.GearCmd,Vcu.Cltch1Cmd,Diff.DiffrntlPrsCmd
  First Order Hold1 : FirstOrderHold  ErrorTolerance=inf
  Rate Transition : RateTransition  InitialCondition=CtrlTcuInitGear
  Rate Transition1 : RateTransition  InitialCondition=CtrlVcuCltch1InitCmd
  GearCmd : Outport  VectorParamsAs1DForOutWhenUnconnected=off
  Cltch1Cmd : Outport  Port=2  VectorParamsAs1DForOutWhenUnconnected=off
  DiffrntlPrsCmd : Outport  Port=3  VectorParamsAs1DForOutWhenUnconnected=off
  wires:
  Cntrl/1 -> Bus Selector3/1
  Bus Selector3/1 -> Rate Transition/1  "<GearCmd>"
  Bus Selector3/3 -> First Order Hold1/1  "<DiffrntlPrsCmd>"
  Bus Selector3/2 -> Rate Transition1/1  "<Cltch1Cmd>"
  Rate Transition1/1 -> Cltch1Cmd/1
  First Order Hold1/1 -> DiffrntlPrsCmd/1
  Rate Transition/1 -> GearCmd/1

== system VirtualVehicleTemplate/Vehicle/Drivetrain Output ==
  AxlTrq : Inport
  EngSpd : Inport  Port=2
  DriveshftSpd : Inport  Port=3
  EMSpd : Inport  Port=4
  TransInfo : Inport  Port=5
  Bus Creator1 : BusCreator  Inputs=5
  Driveline : Outport  VectorParamsAs1DForOutWhenUnconnected=off
  wires:
  Bus Creator1/1 -> Driveline/1  "Driveline"
  DriveshftSpd/1 -> Bus Creator1/3  "DriveshftSpd"
  AxlTrq/1 -> Bus Creator1/1  "AxlTrq"
  EngSpd/1 -> Bus Creator1/2  "EngSpd"
  EMSpd/1 -> Bus Creator1/4  "EMSpd"
  TransInfo/1 -> Bus Creator1/5  "TransInfo"

== system VirtualVehicleTemplate/Vehicle/Electrical System Input ==
  Cntrl : Inport
  Env : Inport  Port=2
  Bus Selector : BusSelector  OutputSignals=Temp
  Bus Selector2 : BusSelector  OutputSignals=Vcu.EMTrqCmd,Vcu.FuelCellCurrCmd,Vcu.FuelCellTempCmd,BMS
  First Order Hold : FirstOrderHold  ErrorTolerance=inf  AllowContinuousInput=on
  First Order Hold1 : FirstOrderHold  ErrorTolerance=inf  AllowContinuousInput=on
  First Order Hold2 : FirstOrderHold  ErrorTolerance=inf  AllowContinuousInput=on
  EMTrqCmd : Outport  VectorParamsAs1DForOutWhenUnconnected=off
  AmbTemp : Outport  Port=2  VectorParamsAs1DForOutWhenUnconnected=off
  FuelCellCurrCmd : Outport  Port=3  VectorParamsAs1DForOutWhenUnconnected=off
  FuelCellTempCmd : Outport  Port=4  VectorParamsAs1DForOutWhenUnconnected=off
  BMS : Outport  Port=5  VectorParamsAs1DForOutWhenUnconnected=off
  wires:
  Env/1 -> Bus Selector/1
  Bus Selector/1 -> AmbTemp/1  "<Temp>"
  Cntrl/1 -> Bus Selector2/1
  Bus Selector2/1 -> First Order Hold/1  "<EMTrqCmd>"
  First Order Hold/1 -> EMTrqCmd/1  "EMTrqCmd"
  First Order Hold1/1 -> FuelCellCurrCmd/1  "FuelCellCurrCmd"
  First Order Hold2/1 -> FuelCellTempCmd/1  "FuelCellTempCmd"
  Bus Selector2/2 -> First Order Hold1/1  "<FuelCellCurrCmd>"
  Bus Selector2/3 -> First Order Hold2/1  "<FuelCellTempCmd>"
  Bus Selector2/4 -> BMS/1  "<BMS>"

== system VirtualVehicleTemplate/Vehicle/Electrical System Output ==
  Battery : Inport
  ElecMachine : Inport  Port=2
  FuelCell : Inport  Port=3
  Out Bus Element4 : Outport  PortName=BatteryFdbk
  Out Bus Element1 : Outport  Port=2  PortName=ElecMachineFdbk
  Out Bus Element2 : Outport  Port=3  PortName=FuelCellFdbk
  wires:
  Battery/1 -> Out Bus Element4/1
  ElecMachine/1 -> Out Bus Element1/1
  FuelCell/1 -> Out Bus Element2/1

== system VirtualVehicleTemplate/Vehicle/Engine Input ==
  Cntrl : Inport
  Bus Creator : BusCreator  Inputs=17
  Bus Selector : BusSelector  OutputSignals=Engine.ThrPosPctCmd,Engine.WgAreaPctCmd,Engine.InjPw,Engine.FuelMainSoi,Engine.SpkAdv,Engine.IntkCamPhaseCmd,Engine.ExhCamPhaseCmd,Engine.TurboRackPosCmd,Engine.EgrVlvAreaPctCmd,Engine.VarCompRatioPosCmd,Engine.IntkVlvLiftCmd,Engine.VarIntkRunLenCmd,Engine.ClsdLpFuelMult,Engine.IntkSwirlVlvPosCmd,Engine.TrqCmd,Engine.LoadCmd,Engine.EstIntkPortFlw
  First Order Hold{,1..16} (17 alike) : FirstOrderHold  ErrorTolerance=inf
  Engine : Outport
  wires:
  Bus Selector/14 -> First Order Hold14/1  "<IntkSwirlVlvPosCmd>"
  Bus Selector/12 -> First Order Hold13/1  "<VarIntkRunLenCmd>"
  Bus Selector/15 -> First Order Hold2/1  "<TrqCmd>"
  Bus Selector/13 -> First Order Hold/1  "<ClsdLpFuelMult>"
  Bus Selector/7 -> First Order Hold8/1  "<ExhCamPhaseCmd>"
  First Order Hold11/1 -> Bus Creator/10  "VarCompRatioPosCmd"
  Bus Selector/4 -> First Order Hold3/1  "<FuelMainSoi>"
  Bus Selector/8 -> First Order Hold9/1  "<TurboRackPosCmd>"
  Bus Selector/5 -> First Order Hold4/1  "<SpkAdv>"
  Bus Selector/9 -> First Order Hold10/1  "<EgrVlvAreaPctCmd>"
  Bus Selector/11 -> First Order Hold12/1  "<IntkVlvLiftCmd>"
  First Order Hold/1 -> Bus Creator/13  "ClsdLpFuelMult"
  Bus Selector/6 -> First Order Hold7/1  "<IntkCamPhaseCmd>"
  First Order Hold1/1 -> Bus Creator/3  "InjPw"
  First Order Hold7/1 -> Bus Creator/6  "IntkCamPhaseCmd"
  First Order Hold9/1 -> Bus Creator/8  "TurboRackPosCmd"
  Bus Selector/3 -> First Order Hold1/1  "<InjPw>"
  First Order Hold5/1 -> Bus Creator/1  "ThrPosPctCmd"
  First Order Hold3/1 -> Bus Creator/4  "FuelMainSoi"
  First Order Hold10/1 -> Bus Creator/9  "EgrVlvAreaPctCmd"
  First Order Hold12/1 -> Bus Creator/11  "IntkVlvLiftCmd"
  First Order Hold13/1 -> Bus Creator/12  "VarIntkRunLenCmd"
  First Order Hold2/1 -> Bus Creator/15  "TrqCmd"
  Bus Selector/1 -> First Order Hold5/1  "<ThrPosPctCmd>"
  Bus Selector/2 -> First Order Hold6/1  "<WgAreaPctCmd>"
  First Order Hold8/1 -> Bus Creator/7  "ExhCamPhaseCmd"
  First Order Hold6/1 -> Bus Creator/2  "WgAreaPctCmd"
  First Order Hold14/1 -> Bus Creator/14  "IntkSwirlVlvPosCmd"
  First Order Hold4/1 -> Bus Creator/5  "SpkAdv"
  Bus Selector/10 -> First Order Hold11/1  "<VarCompRatioPosCmd>"
  Bus Creator/1 -> Engine/1  "Engine"
  Cntrl/1 -> Bus Selector/1
  Bus Selector/16 -> First Order Hold15/1  "<LoadCmd>"
  Bus Selector/17 -> First Order Hold16/1  "<EstIntkPortFlw>"
  First Order Hold15/1 -> Bus Creator/16  "LoadCmd"
  First Order Hold16/1 -> Bus Creator/17  "EstIntkPortFlw"

== system VirtualVehicleTemplate/Vehicle/Engine Output ==
  "EngFdbk " : Inport
  EngFdbk : Outport  VectorParamsAs1DForOutWhenUnconnected=off
  wires:
  "EngFdbk "/1 -> EngFdbk/1  "EngFdbk"

== system VirtualVehicleTemplate/Vehicle/Pedal Cluster Input ==
  Driver : Inport
  Bus Selector : BusSelector  OutputSignals=SteerCmd,AccelCmd,DecelCmd,GearCmd,IgnSwtch
  SteerCmd : Outport  VectorParamsAs1DForOutWhenUnconnected=off
  AccelCmd : Outport  Port=2  VectorParamsAs1DForOutWhenUnconnected=off
  DecelCmd : Outport  Port=3  VectorParamsAs1DForOutWhenUnconnected=off
  DrvrGearCmd : Outport  Port=4  VectorParamsAs1DForOutWhenUnconnected=off
  IgnCmd : Outport  Port=5  VectorParamsAs1DForOutWhenUnconnected=off
  wires:
  Bus Selector/2 -> AccelCmd/1  "<AccelCmd>"
  Driver/1 -> Bus Selector/1
  Bus Selector/3 -> DecelCmd/1  "<DecelCmd>"
  Bus Selector/4 -> DrvrGearCmd/1  "<GearCmd>"
  Bus Selector/1 -> SteerCmd/1  "<SteerCmd>"
  Bus Selector/5 -> IgnCmd/1  "<IgnSwtch>"

== system VirtualVehicleTemplate/Vehicle/Pedal Cluster Output ==
  Driver : Inport
  OperatorFdbk : Outport
  wires:
  Driver/1 -> OperatorFdbk/1

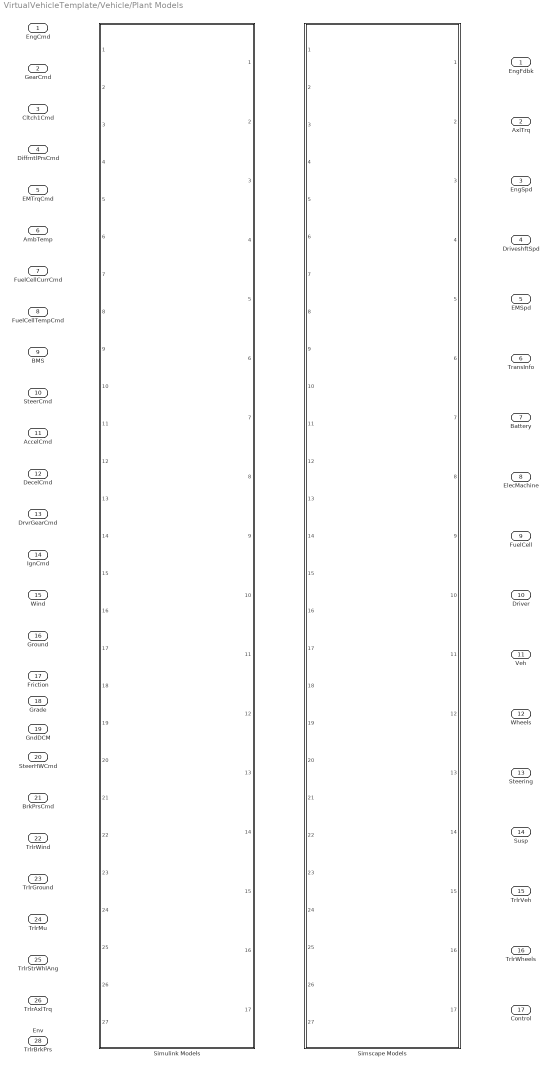
== system VirtualVehicleTemplate/Vehicle/Plant Models ==
  EngCmd : Inport
  GearCmd : Inport  Port=2
  Cltch1Cmd : Inport  Port=3
  DiffrntlPrsCmd : Inport  Port=4
  EMTrqCmd : Inport  Port=5
  AmbTemp : Inport  Port=6
  FuelCellCurrCmd : Inport  Port=7
  FuelCellTempCmd : Inport  Port=8
  BMS : Inport  Port=9
  SteerCmd : Inport  Port=10
  AccelCmd : Inport  Port=11
  DecelCmd : Inport  Port=12
  DrvrGearCmd : Inport  Port=13
  IgnCmd : Inport  Port=14
  Wind : Inport  Port=15
  Ground : Inport  Port=16
  Friction : Inport  Port=17
  Grade : Inport  Port=18
  GndDCM : Inport  Port=19
  SteerHWCmd : Inport  Port=20
  BrkPrsCmd : Inport  Port=21
  TrlrWind : Inport  Port=22
  TrlrGround : Inport  Port=23
  TrlrMu : Inport  Port=24
  TrlrStrWhlAng : Inport  Port=25
  TrlrAxlTrq : Inport  Port=26
  TrlrBrkPrs : Inport  Port=27
  Env : Inport  Port=28
  Simscape Models : Subsystem  VariantControl=SimscapeModels  ReferencedSubsystem=SimscapePlantModels
  Simulink Models : Subsystem  VariantControl=SimulinkModels  ReferencedSubsystem=SimulinkPlantModels
  EngFdbk : Outport
  AxlTrq : Outport  Port=2
  EngSpd : Outport  Port=3
  DriveshftSpd : Outport  Port=4
  EMSpd : Outport  Port=5
  TransInfo : Outport  Port=6
  Battery : Outport  Port=7
  ElecMachine : Outport  Port=8
  FuelCell : Outport  Port=9
  Driver : Outport  Port=10
  Veh : Outport  Port=11
  Wheels : Outport  Port=12
  Steering : Outport  Port=13
  Susp : Outport  Port=14
  TrlrVeh : Outport  Port=15
  TrlrWheels : Outport  Port=16
  Control : Outport  Port=17

== system VirtualVehicleTemplate/Vehicle/Sensor Input ==
  EnvIn : Inport
  Env : Outport
  wires:
  EnvIn/1 -> Env/1  "Env"

== system VirtualVehicleTemplate/Vehicle/Sensor Output ==
  Control : Inport
  CntrlFdbk : Outport
  wires:
  Control/1 -> CntrlFdbk/1

== system VirtualVehicleTemplate/Vehicle/Trailer Input ==
  Env : Inport
  Cntrl : Inport  Port=2
  Bus Selector2 : BusSelector  OutputSignals=Wind
  Bus Selector4 : BusSelector  OutputSignals=Vcu.VcuTrlrBrkPrsCmd
  Constant1 : Constant  Value=zeros(2,1)
  Constant2 : Constant  Value=ones(2,1)
  Constant3 : Constant  Value=[0 0 0 0 0 0]
  Constant4 : Constant  Value=0
  Ground Info Trailer : Subsystem  Commented=on  Variant=on  VariantControlMode=label  VariantControl=Choice  LabelModeActiveChoice=0
  Terminator1 : Terminator
  Terminator2 : Terminator
  TrlrWind : Outport  VectorParamsAs1DForOutWhenUnconnected=off
  TrlrGnd : Outport  Port=2  VectorParamsAs1DForOutWhenUnconnected=off
  TrlrMu : Outport  Port=3  VectorParamsAs1DForOutWhenUnconnected=off
  TrlrStrWhlAng : Outport  Port=4  VectorParamsAs1DForOutWhenUnconnected=off
  TrlrAxlTrq : Outport  Port=5  VectorParamsAs1DForOutWhenUnconnected=off
  TrlrBrkPrs : Outport  Port=6  VectorParamsAs1DForOutWhenUnconnected=off
  wires:
  Bus Selector2/1 -> TrlrWind/1  "<Wind>"
  Env/1 -> Bus Selector2/1, Ground Info Trailer/1(Env)
  Constant3/1 -> TrlrStrWhlAng/1
  Constant4/1 -> TrlrAxlTrq/1
  Bus Selector4/1 -> TrlrBrkPrs/1  "<VcuTrlrBrkPrsCmd>"
  Cntrl/1 -> Bus Selector4/1
  Constant2/1 -> TrlrMu/1
  Constant1/1 -> TrlrGnd/1
  Ground Info Trailer/1(Ground) -> Terminator1/1
  Ground Info Trailer/2(Friction) -> Terminator2/1

== system VirtualVehicleTemplate/Vehicle/Trailer Output ==
  Veh : Inport
  Wheels : Inport  Port=2
  Out Bus Element4 : Outport  PortName=VehFdbk
  Out Bus Element1 : Outport  Port=2  PortName=WheelsFdbk
  wires:
  Wheels/1 -> Out Bus Element1/1
  Veh/1 -> Out Bus Element4/1

== system VirtualVehicleTemplate/Visualization/DataLogging ==
  VehFdbk : Inport
  Bus Selector : BusSelector  OutputSignals=Driver.SteerFdbk
  Terminator : Terminator
  wires:
  VehFdbk/1 -> Bus Selector/1
  Bus Selector/1 -> Terminator/1  "<SteerFdbk>"

== system VirtualVehicleTemplate/Visualization/Emission Calculations ==
  VehSpd : Inport
  TP HC Mass Flow : Inport  Port=2
  TP CO Mass Flow : Inport  Port=3
  TP NOx Mass Flow : Inport  Port=4
  TP CO2 Mass Flow : Inport  Port=5
  Integrator{,1..4} (5 alike) : Integrator
  Kg to g : Gain  Gain=1000
  "Kg to g " : Gain  Gain=1000
  "Kg to g  " : Gain  Gain=1000
  "Kg to g   " : Gain  Gain=1000
  L/100 Km Calc{,1..3} (4 alike) : Product  Inputs=/*
  Rate Transition{,1..3} (4 alike) : RateTransition  Deterministic=off
  Saturation : Saturate  UpperLimit=Inf  LowerLimit=0.2  ZeroCross=off
  Saturation1 : Saturate  UpperLimit=Inf  LowerLimit=1  ZeroCross=off
  Signal Specification5 : SignalSpecification  Unit=m/s
  Unit Conversion5 : UnitConversion
  m to km : Gain  Gain=0.001
  m to mi : Gain  Gain=0.000621371
  TP HC Mass : Outport  VectorParamsAs1DForOutWhenUnconnected=off
  TP CO Mass : Outport  Port=2  VectorParamsAs1DForOutWhenUnconnected=off
  TP NOx Mass : Outport  Port=3  VectorParamsAs1DForOutWhenUnconnected=off
  TP CO2 Mass : Outport  Port=4  VectorParamsAs1DForOutWhenUnconnected=off
  wires:
  L/100 Km Calc/1 -> Rate Transition/1
  m to mi/1 -> Saturation/1
  Saturation/1 -> L/100 Km Calc2/1, L/100 Km Calc1/1, L/100 Km Calc/1
  TP HC Mass Flow/1 -> Integrator1/1
  Integrator1/1 -> Kg to g/1
  Integrator/1 -> m to km/1, m to mi/1
  Kg to g/1 -> L/100 Km Calc/2
  TP CO Mass Flow/1 -> Integrator2/1
  Integrator2/1 -> "Kg to g "/1
  "Kg to g "/1 -> L/100 Km Calc1/2
  TP NOx Mass Flow/1 -> Integrator3/1
  Integrator3/1 -> "Kg to g  "/1
  "Kg to g  "/1 -> L/100 Km Calc2/2
  L/100 Km Calc1/1 -> Rate Transition1/1
  L/100 Km Calc2/1 -> Rate Transition2/1
  TP CO2 Mass Flow/1 -> Integrator4/1
  Integrator4/1 -> "Kg to g   "/1
  "Kg to g   "/1 -> L/100 Km Calc3/2
  L/100 Km Calc3/1 -> Rate Transition3/1
  Saturation1/1 -> L/100 Km Calc3/1
  m to km/1 -> Saturation1/1
  Rate Transition/1 -> TP HC Mass/1  "TP HC Mass (g/mi)"
  Rate Transition1/1 -> TP CO Mass/1  "TP CO Mass (g/mi)"
  Rate Transition2/1 -> TP NOx Mass/1  "TP NOx Mass (g/mi)"
  Rate Transition3/1 -> TP CO2 Mass/1  "TP CO2 Mass (g/km)"
  Unit Conversion5/1 -> Signal Specification5/1
  VehSpd/1 -> Unit Conversion5/1
  Signal Specification5/1 -> Integrator/1

== system VirtualVehicleTemplate/Visualization/ISO 15037-1:2006 ==
  VehFdbk : Inport
  Disabled : Subsystem  VariantControl=0
  Enabled : Subsystem  VariantControl=1

== system VirtualVehicleTemplate/Visualization/Performance Calculations ==
  VehSpd : Inport
  FuelVolFlow : Inport  Port=2
  BattPwr : Inport  Port=3
  Add : Sum
  Divide : Product  Inputs=*/
  Divide1 : Product  Inputs=*/
  Divide2 : Product  Inputs=*/
  Integrator : Integrator
  Integrator1 : Integrator
  L/100 Km Calc : Product  Inputs=/*
  Product : Product
  Rate Transition3 : RateTransition  Deterministic=off
  Saturation : Saturate  UpperLimit=Inf  LowerLimit=0.001  ZeroCross=off
  Saturation1 : Saturate  UpperLimit=Inf  LowerLimit=1e-3  ZeroCross=off
  Signal Specification5 : SignalSpecification  Unit=m/s
  Sqrt : Sqrt
  US EPA kwh/USgal equivalent : Constant  Value=33.7
  US MPG Calc : Product  Inputs=*/
  Unit Conversion5 : UnitConversion
  m to 100Km : Gain  Gain=1/1000/100
  m to mile : Gain  Gain=0.000621371
  m^3 per gal : Gain  Gain=0.00378541
  m^3 to L : Gain  Gain=1000
  m^3 to US Gal : Gain  Gain=264.172
  s per h : Constant  Value=3600
  w per kw : Constant  Value=1000
  US MPG : Outport  VectorParamsAs1DForOutWhenUnconnected=off
  L/100Km : Outport  Port=2  VectorParamsAs1DForOutWhenUnconnected=off
  wires:
  m^3 to US Gal/1 -> Saturation1/1
  m^3 to L/1 -> L/100 Km Calc/2
  Integrator/1 -> m to mile/1, m to 100Km/1
  m to mile/1 -> US MPG Calc/1
  FuelVolFlow/1 -> Add/1
  Integrator1/1 -> m^3 to US Gal/1, m^3 to L/1
  Saturation/1 -> L/100 Km Calc/1
  m to 100Km/1 -> Saturation/1
  L/100 Km Calc/1 -> L/100Km/1  "L/100Km"
  US MPG Calc/1 -> Rate Transition3/1
  Saturation1/1 -> US MPG Calc/2
  Rate Transition3/1 -> US MPG/1  "US MPG"
  w per kw/1 -> Divide/2
  Divide/1 -> Divide2/1
  Divide2/1 -> Divide1/1
  s per h/1 -> Divide1/2
  Divide1/1 -> m^3 per gal/1
  Add/1 -> Integrator1/1
  m^3 per gal/1 -> Add/2
  US EPA kwh/USgal equivalent/1 -> Divide2/2
  BattPwr/1 -> Divide/1
  Sqrt/1 -> Integrator/1
  Product/1 -> Sqrt/1
  Signal Specification5/1 -> Product/2, Product/1
  Unit Conversion5/1 -> Signal Specification5/1
  VehSpd/1 -> Unit Conversion5/1

== system VirtualVehicleTemplate/Visualization/Scope Type ==
  "VehFdbk " : Inport
  "Vis " : Inport  Port=2
  DLC : Subsystem  VariantControl=1
  None : Subsystem  VariantControl=0
  XYZ : Subsystem  VariantControl=2
  " Ref" : Outport  VectorParamsAs1DForOutWhenUnconnected=off

== system VirtualVehicleTemplate/Visualization/Vehicle XY Plotter ==
  "VehFdbk " : Inport
  "Ref " : Inport  Port=2
  Disabled : Subsystem  VariantControl=2
  XY View : Subsystem  VariantControl=0
  XY View Ref : Subsystem  VariantControl=1

== system VirtualVehicleTemplate/Controllers/Active Differential Control (ACD)/No Control ==
  axayaz : Inport
  Steer : Inport  Port=2
  Constant : Constant  Value=0  SampleTime=10/1000
  Constant1 : Constant  Value=0  SampleTime=10/1000
  Terminator : Terminator
  Terminator1 : Terminator
  Vector Concatenate2 : Concatenate  NumInputs=4
  DiffrntlPrsCmd : Outport  VectorParamsAs1DForOutWhenUnconnected=off
  DiffrntlTrqCmd : Outport  Port=2  VectorParamsAs1DForOutWhenUnconnected=off
  wires:
  Constant/1 -> Vector Concatenate2/1, Vector Concatenate2/4, Vector Concatenate2/3, Vector Concatenate2/2
  Steer/1 -> Terminator1/1
  Vector Concatenate2/1 -> DiffrntlPrsCmd/1  "DiffPrsCmd"
  axayaz/1 -> Terminator/1
  Constant1/1 -> DiffrntlTrqCmd/1  "TrqCmd"

== system VirtualVehicleTemplate/Controllers/Battery Management System (BMS)/No BMS ==
  Bus Creator : BusCreator  Inputs=1
  Bus Creator1 : BusCreator  Inputs=1
  Bus Creator3 : BusCreator  Inputs=1
  Bus Creator4 : BusCreator  Inputs=2
  Constant : Constant  Value=0  SampleTime=-1
  Constant1 : Constant  Value=0  SampleTime=-1
  Constant2 : Constant  Value=0  SampleTime=-1
  BMSInfo : Outport
  BMSCmd : Outport  Port=2
  wires:
  Bus Creator/1 -> BMSInfo/1  "BMSInfo"
  Bus Creator1/1 -> Bus Creator/1  "SOC"
  Constant/1 -> Bus Creator1/1  "SOC_CC"
  Bus Creator3/1 -> BMSCmd/1  "BMSCmd"
  Bus Creator4/1 -> Bus Creator3/1  "CurrentLimitsBus"
  Constant1/1 -> Bus Creator4/1  "DischargeCurrentLimit"
  Constant2/1 -> Bus Creator4/2  "ChargeCurrentLimit"
